simulink model "trajetorianominalSimulink"  (R2019a)
settings: Solver=VariableStepAuto  StartTime=0.0  StopTime=170  RelTol=1e-3
undefined symbols (not defined in the file): A, B
settings Model: Creator=Cliente  LastModifiedBy=Cliente

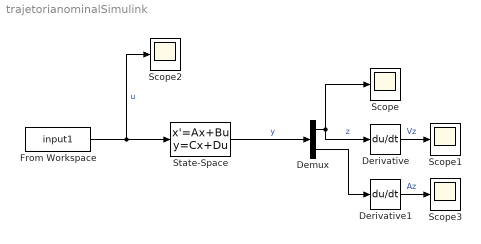
== system trajetorianominalSimulink ==
  Demux : Demux  Outputs=2
  Derivative : Derivative
  Derivative1 : Derivative
  From Workspace : FromWorkspace  VariableName=input1  SampleTime=0
  Scope{,1..3} (4 alike) : Scope
  State-Space : StateSpace  A=A  B=B  C=[1 0;0 1]  D=[0;0]  InitialCondition=[0; 0]
  wires:
  Derivative/1 -> Scope1/1  "Vz"
  Demux/1 -> Scope/1, Derivative/1  "z"
  Demux/2 -> Derivative1/1
  Derivative1/1 -> Scope3/1  "Az"
  State-Space/1 -> Demux/1  "y"
  From Workspace/1 -> State-Space/1, Scope2/1  "u"
